simulink model "questao28_sim"  (R2020b)
settings: Solver=VariableStepAuto  StartTime=0.0  StopTime=300  RelTol=1e-3
settings Model: Creator=lucas  LastModifiedBy=lucas

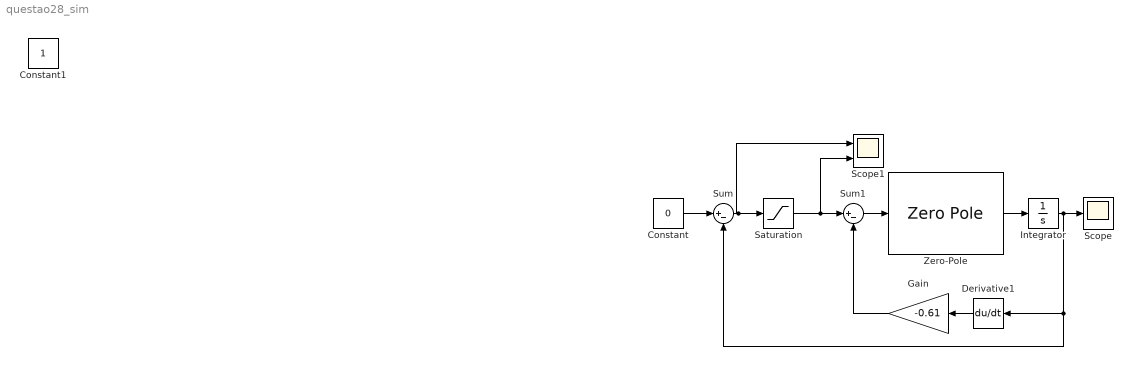
== system questao28_sim ==
  Constant : Constant  Value=0
  Derivative1 : Derivative  CoefficientInTFapproximation=0
  Gain : Gain  Gain=-0.61
  Integrator : Integrator  InitialCondition=1
  Saturation : Saturate
  Scope : Scope
  Scope1 : Scope  NumInputPorts=2
  Sum : Sum  Inputs=|+-
  Sum1 : Sum  Inputs=|+-
  Zero-Pole : ZeroPole  Zeros=[]  Poles=[-1 -4]  Gain=5
  Constant1 : Constant  IOType=siggen
  wires:
  Constant/1 -> Sum/1
  Sum/1 -> Scope1/1, Saturation/1
  Saturation/1 -> Scope1/2, Sum1/1
  Sum1/1 -> Zero-Pole/1
  Gain/1 -> Sum1/2
  Derivative1/1 -> Gain/1
  Zero-Pole/1 -> Integrator/1
  Integrator/1 -> Derivative1/1, Sum/2, Scope/1
